simulink model "model"  (Simulink 8.7)
settings: Solver=ode45  StartTime=0.0  StopTime=25  RelTol=1e-3
undefined symbols (not defined in the file): h, sigbuilder_block
libraries: simulink x1
settings Model: Creator=Krzys  LastModifiedBy=student
settings DataIOCC: SignalLoggingSaveFormat=ModelDataLogs
settings DebuggingCC: SolverPrmCheckMsg=warning  FcnCallInpInsideContextMsg=UseLocalSettings  StateNameClashWarn=warning
settings GRTTargetCC: GeneratePreprocessorConditionals=Use local settings  CombineOutputUpdateFcns=off  GRTInterface=on

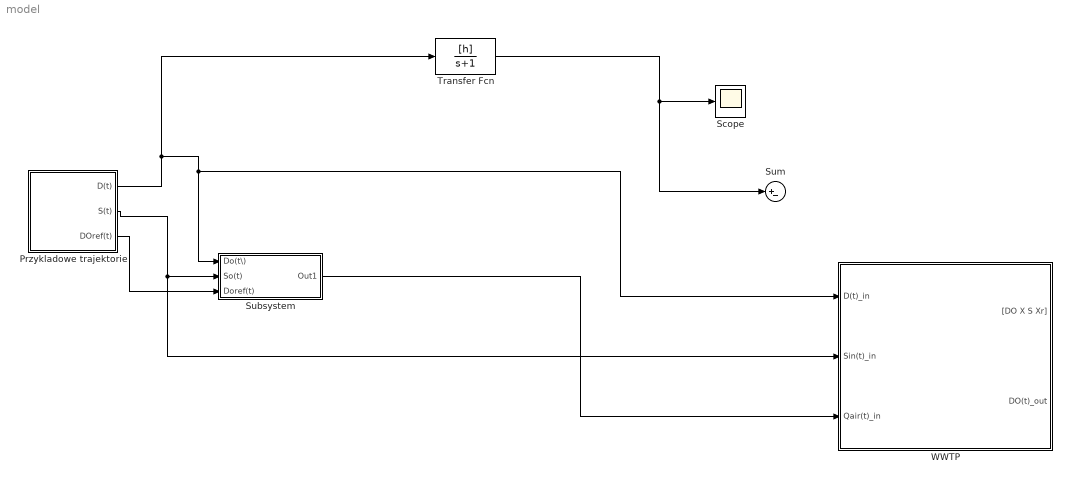
== system model ==
  Przykladowe trajektorie : Subsystem  Tag=STV Subsys  LoadFcn=sigbuilder_block('load');  StartFcn=sigbuilder_block('start');  StopFcn=sigbuilder_block('stop');  ClipboardFcn=sigbuilder_block('clipboard');  mask(Sigbuilder block){}
      mask help: Sigbuilder GUI
      mask init:
      | if ~strcmp(get_param(bdroot(gcbh),'SimulationStatus'),'stopped') tuvar = sigbuilder_block('maskInit'); end
      settings: CopyFcn=sigbuilder_block('copy');  DeleteFcn=sigbuilder_block('delete');  ModelCloseFcn=sigbuilder_block('modelClose');  PreSaveFcn=sigbuilder_block('preSave');  PauseFcn=sigbuilder_block('pause')  ContinueFcn=sigbuilder_block('continue')  NameChangeFcn=sigbuilder_block('namechange');  OpenFcn=sigbuilder_block('open',[356.25 132.75 550.5 399.75 ]);  CloseFcn=sigbuilder_block('close');
      mask Display: plot(0,0,100,100,[10,10,40,40,10],[80,20,20,80,80],[40,10],[50,50], [40,27,10],[65,72,56],[40,25,25,10],[28,28,43,43]);
  Scope : Scope
  Subsystem : Subsystem
  Sum : Sum  Inputs=|+-
  Transfer Fcn : TransferFcn  Numerator=[h]  Denominator=[1 1]
  WWTP : Subsystem  mask{stateX=1225, stateS=20, stateDO=6, stateXr=2333}
  wires:
  Przykladowe trajektorie/1(D(t)) -> Transfer Fcn/1, Subsystem/1(Do(t\)), WWTP/1(D(t)_in)
  Przykladowe trajektorie/2(S(t)) -> Subsystem/2("So(t) "), WWTP/2(Sin(t)_in)
  Transfer Fcn/1 -> Sum/1, Scope/1
  Przykladowe trajektorie/3(DOref(t)) -> Subsystem/3("Doref(t) ")
  Subsystem/1(Out1) -> WWTP/3(Qair(t)_in)

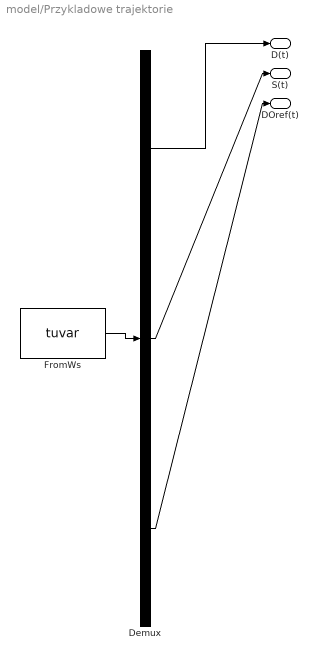
== system model/Przykladowe trajektorie ==
  Demux : Demux  Tag=STV Demux  Outputs=3
  FromWs : FromWorkspace  Tag=STV FromWs  VariableName=tuvar  SampleTime=0  SigBuilderData=DataTag0  VnvData=DataTag1
      SigBuilderData=|
      | common.afterFinalStr = 'Extrapolate'
      | common.sampleTime = 0
      | dataSet.timeRange = [0 24]
      | dataSet.name = 'Group 1'
      | sbobj.Groups.Name = 'Group 1'
      | sbobj.Groups.Signals(1).Name = 'D(t)'
      | sbobj.Groups.Signals(1).XData = [0 4 4 7 7 12 12 16 16 20 20 24]
      | sbobj.Groups.Signals(1).YData = [0.065 0.065 0.025 0.025 0.05 0.05 0.04 0.04 0.065 0.065 0.03 0.03]
      | sbobj.Groups.Signals(2).Name = 'S(t)'
      | sbobj.Groups.Signals(2).XData = [0 4 4 7 7 12 12 16 16 20 20 24]
      | sbobj.Groups.Signals(2).YData = [600 600 200 200 500 500 400 400 600 600 350 350]
      | sbobj.Groups.Signals(3).Name = 'DOref(t)'
      | sbobj.Groups.Signals(3).XData = [0 2 2 4 4 6 6 8 8 10 10 12 12 14 14 16 16 18 18 20 20 22 22 24]
      | sbobj.Groups.Signals(3).YData = [1.5 1.5 9.4 9.4 5 5 2 2 2.5 2.5 7 7 2.5 2.5 4 4 8.5 8.5 6 6 2 2 3 3]
      | sbobj.Groups.TimeRange = [0 24]
  D(t) : Outport  Tag=STV Outport
  S(t) : Outport  Tag=STV Outport  Port=2
  DOref(t) : Outport  Tag=STV Outport  Port=3
  wires:
  Demux/1 -> D(t)/1
  FromWs/1 -> Demux/1
  Demux/2 -> S(t)/1
  Demux/3 -> DOref(t)/1

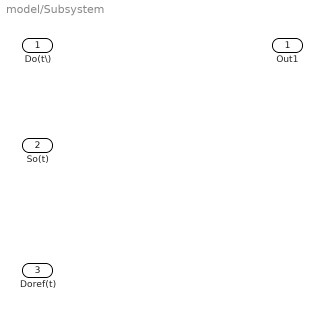
== system model/Subsystem ==
  Do(t\) : Inport
  "So(t) " : Inport  Port=2
  "Doref(t) " : Inport  Port=3
  Out1 : Outport

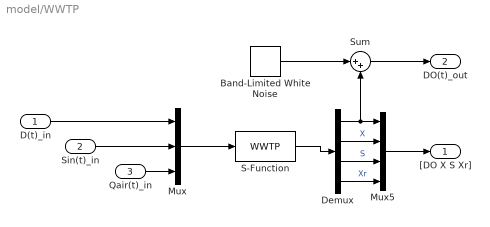
== system model/WWTP ==
  D(t)_in : Inport
  Sin(t)_in : Inport  Port=2
  Qair(t)_in : Inport  Port=3
  Band-Limited White Noise : simulink/Sources/Band-Limited White Noise  Cov=[0.001]  Ts=1/60  seed=[23341]
  Demux : Demux
  Mux : Mux  Inputs=3
  Mux5 : Mux
  S-Function : S-Function  FunctionName=WWTP  Parameters=stateX stateS stateDO stateXr  SFunctionDeploymentMode=off  EnableBusSupport=off
  Sum : Sum  Inputs=|++
  "[DO X S Xr]" : Outport
  DO(t)_out : Outport  Port=2
  wires:
  Mux5/1 -> "[DO X S Xr]"/1
  D(t)_in/1 -> Mux/1
  Sin(t)_in/1 -> Mux/2
  Qair(t)_in/1 -> Mux/3
  Mux/1 -> S-Function/1
  S-Function/1 -> Demux/1
  Demux/2 -> Mux5/2  "X"
  Demux/3 -> Mux5/3  "S"
  Demux/4 -> Mux5/4  "Xr"
  Demux/1 -> Mux5/1, Sum/2
  Band-Limited White Noise/1 -> Sum/1
  Sum/1 -> DO(t)_out/1
